simulink library "SimscapeCustomComponents_lib"  (R2025b)
settings: Solver=VariableStepAuto  StartTime=0.0  StopTime=10.0  RelTol=1e-3
undefined symbols (not defined in the file or in its folder): base, baseVdc, capacity, DiscIntNeverNeededParam, ee_sli_rtmsupport, filterInductance, freqeuncy, frequency, gcbh, gflInverter, gfmInverter, iMaxPU, Inertia, initialSOC, plantRating, solar, Ts, ups, Vac, windSystem, windTurbine
libraries: fl_lib x397, nesl_utility x171, eeGeneralControl x85, ee_lib x82, simulink x72, datacenter_lib x68, eeTransforms x38, slpidlib x24, buildingEnergy_lib x20, SimscapeFluids_lib x17, eeSinusoidalMeasurementV2 x8, eePwmGenerator x8
(part 2 of 24)

== system SimscapeCustomComponents_lib/Datacenter/CDU ==
  CDU (LUT) : Subsystem  mask{numPump=2, flowrate_vec=[100:100:1000]/60000, capacity_vec=10000*ones(1,10), effPump_vec=[0.4,0.42,0.45,0.5,0.55,0.6,0.62,0.65,0.65,0.64], prDrop_mat=1000*[0.28,1.11,2.5,4.44,6.94,10,13.61,17.78,22.5,27.78; 5.6,2.22,5,8.88,13.88,20,27.22,35.56,45,55.56]', speed=1}
      mask prompts: numPump "Total number of pumps (-)"; flowrate_vec "Coolant volumetric flowrate vector (m^3/s)"; capacity_vec "Heat exchanger capacity vector (W)"; effPump_vec "Pump efficiency vector, 0-1 (-)"; prDrop_mat "Pressure drop (Pa)"; speed "Pump speed scaling (-)"
      settings: CopyFcn=set_param(gcbh,'LinkStatus','none');  PortSchema="{\"entries\":[{\"content\":{\"sides\":[{\"content\":{\"connectorIds\":[\"LConn1\",\"LConn2\"]},\"type\":\"ConnectorPlacement.EquallySpacedRectSide\",\"uuid\":\"dd9276e8-a048-49df-a05c-f18b45aafce3\"},{\"content\":{\"connectorIds\":[\"RConn1\",\"RConn2\"],\"side\":\"RIGHT\"},\"type\":\"ConnectorPlacement.EquallySpacedRectSide\",\"uuid\":\"f4cbe01b-cfd4-4d60-aff7-a07955033ed5\"},{\"content\":{\"connectorIds\":[\"LConn3\"],\"side\":\"TOP\"},\"type\":\"ConnectorPlacement.EquallySpacedRectSide\",\"uuid\":\"ad27df56-4241-452c-8570-6a66062dd2f2\"}]},\"type\":\"ConnectorPlacement.EquallySpacedConnector\",\"uuid\":\"0333b5f9-1896-45e0-922d-790b0e5dd980\"}],\"packageUris\":[\"http://schema.mathworks.com/mf0/Connector/R2020b\"],\"version\":\"1.0\"}"
      mask Help: web("DocumentationCDULUT.html")
      mask DialogControl Container4 Prompt: CDU
      mask Display: image('icon_CDUtableBased.png');
  CDU (TL) : Subsystem  mask{extFluidMdot=[.3, .5, 1, 1.3, 1.7, 2, 2.6, 3.3], extFluidPrDrop=ones(1,8), extFluidVol=0.01, extFluidPipeArea=0.01, intFluidMdot=[.3, .5, .6, .7, 1, 1.4, 1.9, 2.3], intFluidPrDrop=ones(1,8), intFluidVol=0.01, intFluidPipeArea=0.01, spDissipationTbl=[.324, .3533, .404, .4253, .4333, .4373, .4453, .4533; .3813, .424, .496, .5307, .544, .5547, .5693, .5787; .4267, .4827, .5813, .6173, .6413, .6573, .672, .6827; .4613, .528, .64, .6987, .7267, .7467, .7707, .7853; .5533, .6467, .8227, .928, .9853, 1.0187, 1.0653, 1.0973; .58, .688, .8853, 1.0147, 1.08, 1.124, 1.176, 1.2147; .624, .7467, .992, 1.148, 1.244, 1.304, 1.3773, 1.4267; .656, .7907, 1.0667, 1.26, 1.376, 1.452, 1.548, 1.612], effPipeLen=5, pumpCapacityVec=[0.1:0.1:1.2]/998, pumpRefHeadVec=[239, 238.5, 232, 230, 222, 216, 208, 196, 186, 170,150,130], pumpRefBrkPowVec=[0.3,0.4,0.45,0.5,0.55,0.6,0.65,0.7,0.75,0.78,0.79,0.798], pumpEff=[20,40,50,60,65,70,75,75,75,73,68,60]/100, nPumps=3, speedLimFactor=1, pumpNominalRPM=3500, pumpImpellerDiaFactor=1, iniT=293, iniP=0.101325, refT=293, refP=0.101325, refDensity=998}
      mask prompts: extFluidMdot "External liquid loop mass flow rate vector (kg/s)"; extFluidPrDrop "External liquid loop pressure drop vector (kPa)"; extFluidVol "External liquid volume in heat exchanger (m^3)"; extFluidPipeArea "External liquid loop pipe cross-sectional area (m^2)"; intFluidMdot "Internal liquid loop mass flow rate vector (kg/s)"; intFluidPrDrop "Internal liquid loop pressure drop vector (kPa)"; intFluidVol "Internal liquid volume in heat exchanger (m^3)"; intFluidPipeArea "Internal liquid loop pipe cross-sectional area (m^2)"; spDissipationTbl "Specific dissipation table, SD[mdot_int,mdot_ext] (kW/K)"; effPipeLen "Effective pipe length for rack cooling (m)"; pumpCapacityVec "Reference capacity vector for each pump (m^3/s)"; pumpRefHeadVec "Reference head vector for each pump (m)"; pumpRefBrkPowVec "Reference brake power vector (kW)"; pumpEff "Electrical efficiency vector, 0-1 (-)"; nPumps "Total number of pumps (-)"; speedLimFactor "Pump speed upper limit factor (-)"; pumpNominalRPM "Pump nominal rating (rpm)"; pumpImpellerDiaFactor "Impeller diameter scale factor (-)"; iniT "Initial temperature (K)"; iniP "Initial pressure (MPa)"; refT "Reference flow temperature (K)"; refP "Reference flow pressure (MPa)"; refDensity "Reference density for internal liquid (kg/m^3)"
      settings: CopyFcn=set_param(gcbh,'LinkStatus','none');  PortSchema="{\"entries\":[{\"content\":{\"sides\":[{\"content\":{\"connectorIds\":[\"LConn1\",\"LConn2\",\"LConn3\"]},\"type\":\"ConnectorPlacement.EquallySpacedRectSide\",\"uuid\":\"dd9276e8-a048-49df-a05c-f18b45aafce3\"},{\"content\":{\"connectorIds\":[\"RConn1\",\"RConn2\"],\"side\":\"RIGHT\"},\"type\":\"ConnectorPlacement.EquallySpacedRectSide\",\"uuid\":\"f4cbe01b-cfd4-4d60-aff7-a07955033ed5\"},{\"content\":{\"connectorIds\":[\"LConn4\"],\"side\":\"TOP\"},\"type\":\"ConnectorPlacement.EquallySpacedRectSide\",\"uuid\":\"ad27df56-4241-452c-8570-6a66062dd2f2\"}]},\"type\":\"ConnectorPlacement.EquallySpacedConnector\",\"uuid\":\"0333b5f9-1896-45e0-922d-790b0e5dd980\"}],\"packageUris\":[\"http://schema.mathworks.com/mf0/Connector/R2020b\"],\"version\":\"1.0\"}"
      mask Help: web("DocumentationCDUTL.html")
      mask DialogControl Container5 Prompt: Heat Exchanger
      mask DialogControl Container8 Prompt: Set External Fluid Properties
      mask DialogControl Container7 Prompt: Set Internal Fluid Properties
      mask DialogControl Container9 Prompt: Heat Transfer
      mask DialogControl Container6 Prompt: Pumps
      mask DialogControl Container4 Prompt: Initial Conditions
      mask Display: image('icon_CDUthermalLiquid.png');
  CDU (TL) Detailed : Subsystem  mask{extFluidMdot=[.3, .5, 1, 1.3, 1.7, 2, 2.6, 3.3], extFluidPrDrop=ones(1,8), extFluidVol=0.01, extFluidPipeArea=0.01, intFluidMdot=[.3, .5, .6, .7, 1, 1.4, 1.9, 2.3], intFluidPrDrop=ones(1,8), intFluidVol=0.01, intFluidPipeArea=0.01, spDissipationTbl=[.324, .3533, .404, .4253, .4333, .4373, .4453, .4533; .3813, .424, .496, .5307, .544, .5547, .5693, .5787; .4267, .4827, .5813, .6173, .6413, .6573, .672, .6827; .4613, .528, .64, .6987, .7267, .7467, .7707, .7853; .5533, .6467, .8227, .928, .9853, 1.0187, 1.0653, 1.0973; .58, .688, .8853, 1.0147, 1.08, 1.124, 1.176, 1.2147; .624, .7467, .992, 1.148, 1.244, 1.304, 1.3773, 1.4267; .656, .7907, 1.0667, 1.26, 1.376, 1.452, 1.548, 1.612], pumpCapacityVec=[0.1:0.1:1.2]/998, pumpRefHeadVec=[239, 238.5, 232, 230, 222, 216, 208, 196, 186, 170,150,130], pumpRefBrkPowVec=[0.3,0.4,0.45,0.5,0.55,0.6,0.65,0.7,0.75,0.78,0.79,0.798], pumpEff=[20,40,50,60,65,70,75,75,75,73,68,60]/100, nPumps=3, speedLimFactor=1, pumpNominalRPM=3500, pumpImpellerDiaFactor=1, iniT=293, iniP=0.101325, refT=293, refP=0.101325, refDensity=998}
      mask prompts: extFluidMdot "External liquid loop mass flow rate vector (kg/s)"; extFluidPrDrop "External liquid loop pressure drop vector (kPa)"; extFluidVol "External liquid volume in heat exchanger (m^3)"; extFluidPipeArea "External liquid loop pipe cross-sectional area (m^2)"; intFluidMdot "Internal liquid loop mass flow rate vector (kg/s)"; intFluidPrDrop "Internal liquid loop pressure drop vector (kPa)"; intFluidVol "Internal liquid volume in heat exchanger (m^3)"; intFluidPipeArea "Internal liquid loop pipe cross-sectional area (m^2)"; spDissipationTbl "Specific dissipation table, SD[mdot_int,mdot_ext] (kW/K)"; pumpCapacityVec "Reference capacity vector for each pump (m^3/s)"; pumpRefHeadVec "Reference head vector for each pump (m)"; pumpRefBrkPowVec "Reference brake power vector (kW)"; pumpEff "Electrical efficiency vector, 0-1 (-)"; nPumps "Total number of pumps (-)"; speedLimFactor "Pump speed upper limit factor (-)"; pumpNominalRPM "Pump nominal rating (rpm)"; pumpImpellerDiaFactor "Impeller diameter scale factor (-)"; iniT "Initial temperature (K)"; iniP "Initial pressure (MPa)"; refT "Reference flow temperature (K)"; refP "Reference flow pressure (MPa)"; refDensity "Reference density for internal liquid (kg/m^3)"
      settings: CopyFcn=set_param(gcbh,'LinkStatus','none');  PortSchema="{\"entries\":[{\"content\":{\"sides\":[{\"content\":{\"connectorIds\":[\"LConn1\",\"LConn2\",\"LConn3\"]},\"type\":\"ConnectorPlacement.EquallySpacedRectSide\",\"uuid\":\"f1196858-c1c1-4a92-9579-b8bafb400d5a\"},{\"content\":{\"connectorIds\":[\"RConn1\",\"RConn2\"],\"side\":\"RIGHT\"},\"type\":\"ConnectorPlacement.EquallySpacedRectSide\",\"uuid\":\"0b2555b3-cd40-4e71-81ae-83eafd2a0952\"},{\"content\":{\"connectorIds\":[\"LConn4\",\"LConn5\"],\"side\":\"TOP\"},\"type\":\"ConnectorPlacement.EquallySpacedRectSide\",\"uuid\":\"202bfcad-adb5-4fb7-94c5-4d194a2e1d47\"}]},\"type\":\"ConnectorPlacement.EquallySpacedConnector\",\"uuid\":\"91782cfb-007a-4e62-9f99-de6082fc4e38\"}],\"packageUris\":[\"http://schema.mathworks.com/mf0/Connector/R2020b\"],\"version\":\"1.0\"}"
      mask Help: web("DocumentationCDUTL.html")
      mask DialogControl Container5 Prompt: Heat Exchanger
      mask DialogControl Container8 Prompt: Set External Fluid Properties
      mask DialogControl Container7 Prompt: Set Internal Fluid Properties
      mask DialogControl Container9 Prompt: Heat Transfer
      mask DialogControl Container6 Prompt: Pumps
      mask DialogControl Container4 Prompt: Initial Conditions
      mask Display: image('icon_CDUthermalLiquidDetailed.png');
  Rack Air Cooling : Subsystem  mask{nFans=5, flowVec=[0.1 0.2 0.3 0.4 0.5], prDropVec=[50 100 150 220 280], fanEffVec=[0.58, 0.60, 0.61, 0.60, 0.59], fluidDen=1.28, fluidCp=1005}
      mask prompts: nFans "Number of fans (-)"; flowVec "Fan flow rate vector (m^3/s)"; prDropVec "Pressure drop vector (Pa)"; fanEffVec "Fan efficiency vector (-)"; fluidDen "Fluid density (kg/m^3)"; fluidCp "Fluid heat capacity (J/(Kg*K))"
      settings: CopyFcn=set_param(gcbh,'LinkStatus','none');
      mask Help: web("DocumentationRackAirCooling.html")
      mask DialogControl Container3 Prompt: Fans
      mask DialogControl Container4 Prompt: Fluid Properties
      mask Display: image('icon_PDUfanCooling.png');

== system SimscapeCustomComponents_lib/Datacenter/Facilities ==
  CHB Module (Average Model) : datacenter_lib/CHB Module (Average Model)  OnResistance=1e-3 Ohm  GridVoltage=13800 V  TotalDCVoltage=13200 V  iAC_specify=off  iAC_priority=None  iAC=0 A  iAC_nominal_specify=off  iAC_nominal_value=1  iAC_nominal_unit=A  vAC_specify=off  vAC_priority=None  vAC=0 V  vAC_nominal_specify=off  vAC_nominal_value=1  vAC_nominal_unit=V  iDC_specify=off  iDC_priority=None  iDC=0 A  iDC_nominal_specify=off  iDC_nominal_value=1  iDC_nominal_unit=A  vDC_specify=off  vDC_priority=None  vDC=0 V  vDC_nominal_specify=off  vDC_nominal_value=1  vDC_nominal_unit=V  vOn_specify=off  vOn_priority=None  vOn=0 V  vOn_nominal_specify=off  vOn_nominal_value=1  vOn_nominal_unit=V
      settings: InternalSimscapePortConfiguration="{\"Bottom\":[],\"Left\":[{\"id\":\"m\",\"label\":\"m\",\"type\":\"input\"},{\"id\":\"ACPositive\",\"label\":\"AC+\",\"type\":\"foundation.electrical.electrical\"},{\"id\":\"ACNegative\",\"label\":\"AC-\",\"type\":\"foundation.electrical.electrical\"}],\"Right\":[{\"id\":\"DCPositive\",\"label\":\"DC+\",\"type\":\"foundation.electrical.electrical\"},{\"id\":\"DCNegative\",\"label\":\"DC-\",\"type\":\"foundation.electrical.electrical\"}],\"Top\":[]}"
  CHB Phase Leg (Average Model) : datacenter_lib/CHB Phase Leg (Average Model)  NumModules=3  OnResistance=1e-3 Ohm  InitialDCVoltage=4400 V  GridVoltage=13800 V  TotalDCVoltage=13200 V
      settings: InternalSimscapePortConfiguration="{\"Bottom\":[],\"Left\":[{\"id\":\"ACPositive\",\"label\":\"AC+\",\"type\":\"foundation.electrical.electrical\"},{\"id\":\"ACNegative\",\"label\":\"AC-\",\"type\":\"foundation.electrical.electrical\"},{\"id\":\"m\",\"label\":\"m\",\"type\":\"input\"}],\"Right\":[{\"id\":\"DCPositive\",\"label\":\"DC+\",\"type\":\"foundation.electrical.electrical\"},{\"id\":\"DCNegative\",\"label\":\"DC-\",\"type\":\"foundation.electrical.electrical\"}],\"Top\":[]}"
  Chiller : Subsystem  mask{nominalRating=270, nominalFlowrate=185, nominalPrDrop=0.05, cop=13, volume=1, portArea=0.01, initialP=0.101325, initialT=300}
      mask prompts: nominalRating "Nominal rating (kW)"; nominalFlowrate "Nominal flowrate (kg/s)"; nominalPrDrop "Nominal pressure drop (MPa)"; cop "Coefficient of performance (-)"; volume "Chiller volume (m^3)"; portArea "Cross-sectional port area (m^2)"; initialP "Initial pressure (MPa)"; initialT "Initial temperature (K)"
      settings: CopyFcn=set_param(gcbh,'LinkStatus','none');  PortSchema="{\"entries\":[{\"content\":{\"sides\":[{\"content\":{\"connectorIds\":[\"LConn1\",\"LConn2\"]},\"type\":\"ConnectorPlacement.EquallySpacedRectSide\",\"uuid\":\"7d4232d9-e275-4255-9dc4-bc3f1c69ec46\"},{\"content\":{\"connectorIds\":[\"RConn1\",\"RConn2\"],\"side\":\"RIGHT\"},\"type\":\"ConnectorPlacement.EquallySpacedRectSide\",\"uuid\":\"7ca0ea83-7974-4453-97b6-22bfcf77b4f1\"},{\"content\":{\"connectorIds\":[\"LConn3\",\"LConn4\"],\"side\":\"TOP\"},\"type\":\"ConnectorPlacement.EquallySpacedRectSide\",\"uuid\":\"65c43657-b3f1-43d9-9625-8376acff2e22\"},{\"content\":{\"side\":\"BOTTOM\"},\"type\":\"ConnectorPlacement.EquallySpacedRectSide\",\"uuid\":\"1eb88563-12e2-4927-be7c-afaa658f242e\"}]},\"type\":\"ConnectorPlacement.EquallySpacedConnector\",\"uuid\":\"9af448fb-8903-42ba-af4c-44d5135333f1\"}],\"packageUris\":[\"http://schema.mathworks.com/mf0/Connector/R2020b\"],\"version\":\"1.0\"}"
      mask Help: web('DocumentationChiller.html')
      mask DialogControl Container2 Prompt: Rating
      mask DialogControl Container3 Prompt: Initial Conditions
      mask Display: image('icon_Chiller.png');
  Compute Profile Source (LLM Workload Generator) : datacenter_lib/Compute Profile Source (LLM Workload Generator)  gpuModel=GPUModel.B200  numGPUs=288  workloadType=WorkloadType.Training  timeScale=1  tokenSource=TokenSource.Fixed  showAdvanced=false  customPeakTFLOPS=1000  customHbmBW=4e12 1/s  hbmBW=8e12 1/s  interNodeBW=50e9 1/s  llmSize=LLMModelSize.Llama_70B  customNumParams_B=70  customNumLayers=80  customPrecision=2  parallelism=ParallelismStrategy.TP8_PP4  customTP=8  customPP=4  microBatch=8  globalBatch=2048  seqLength=2048  idleUtil=0.05  fwdUtil=0.85  bwdUtil=0.92  commSyncUtil=0.15  prompt_tokens=512  output_tokens=256  num_concurrent=8  batch_size=8  allreduce_latency=5e-6 s  baseInfUtil=0.08  baseInfFrac=0.10  MFU=0.85  checkpointOverhead=0.03  stragglerOverhead=0.02  trainableParamFrac=0.02  evalInterval=5  evalBatches=2  ft_checkpointOverhead=0.05  enableNoise=true  noiseAmplitude=0.08  stepJitter=0.15  enableFilter=false  filterTimeConstant=0.01 s  t_step_specify=off  t_step_priority=Low  t_step=0 s  t_step_nominal_specify=off  t_step_nominal_value=1  t_step_nominal_unit=s  phase_id_specify=off  phase_id_priority=None  phase_id=0  phase_id_nominal_specify=off  phase_id_nominal_value=1  phase_id_nominal_unit=1  utilization_specify=off  utilization_priority=None  utilization=0  utilization_nominal_specify=off  utilization_nominal_value=1  utilization_nominal_unit=1  step_count_specify=off  step_count_priority=None  step_count=0  step_count_nominal_specify=off  step_count_nominal_value=1  step_count_nominal_unit=1  tc_utilization_specify=off  tc_utilization_priority=None  tc_utilization=0  tc_utilization_nominal_specify=off  tc_utilization_nominal_value=1  tc_utilization_nominal_unit=1  hbm_utilization_specify=off  hbm_utilization_priority=None  hbm_utilization=0  hbm_utilization_nominal_specify=off  hbm_utilization_nominal_value=1  hbm_utilization_nominal_unit=1  tokens_per_sec_obs_specify=off  tokens_per_sec_obs_priority=None  tokens_per_sec_obs=0 1/s  tokens_per_sec_obs_nominal_specify=off  tokens_per_sec_obs_nominal_value=1  tokens_per_sec_obs_nominal_unit=1/s  ttft_obs_specify=off  ttft_obs_priority=None  ttft_obs=0 s  ttft_obs_nominal_specify=off  ttft_obs_nominal_value=1  ttft_obs_nominal_unit=s
      settings: InternalSimscapePortConfiguration="{\"Bottom\":[],\"Left\":[{\"id\":\"prompt_len_in\",\"label\":\"Tn(in)\",\"type\":\"input\"}],\"Right\":[{\"id\":\"compute\",\"label\":\"C\",\"type\":\"output\"},{\"id\":\"U\",\"label\":\"U\",\"type\":\"output\"}],\"Top\":[]}"
  DAB Generalized Average Model : datacenter_lib/DAB Generalized Average Model  N=1  L1=68.2e-6 H  L2=68.2e-6 H  Rt=0.5 Ohm  Co=540e-6 F  fs=10000 Hz  vo0_init=0 V  it1R_init=0 A  it1I_init=0 A  include_esr=false  Rc=0.25 Ohm  i_in_specify=off  i_in_priority=None  i_in=0 A  i_in_nominal_specify=off  i_in_nominal_value=1  i_in_nominal_unit=A  i_out_specify=off  i_out_priority=None  i_out=0 A  i_out_nominal_specify=off  i_out_nominal_value=1  i_out_nominal_unit=A  v_in_specify=off  v_in_priority=None  v_in=0 V  v_in_nominal_specify=off  v_in_nominal_value=1  v_in_nominal_unit=V  v_out_specify=off  v_out_priority=None  v_out=0 V  v_out_nominal_specify=off  v_out_nominal_value=1  v_out_nominal_unit=V
      settings: InternalSimscapePortConfiguration="{\"Bottom\":[],\"Left\":[{\"id\":\"p_in\",\"label\":\"V+\",\"type\":\"foundation.electrical.electrical\"},{\"id\":\"n_in\",\"label\":\"V-\",\"type\":\"foundation.electrical.electrical\"},{\"id\":\"d\",\"label\":\"d\",\"type\":\"input\"}],\"Right\":[{\"id\":\"p_out\",\"label\":\"Vo+\",\"type\":\"foundation.electrical.electrical\"},{\"id\":\"n_out\",\"label\":\"Vo-\",\"type\":\"foundation.electrical.electrical\"}],\"Top\":[]}"
  PSU PFC Stage (Average Model) : datacenter_lib/PSU PFC Stage (Average Model)  C_dc=2e-3 F  V_dc_ref=400 V  Kp_pfc=1.0 W/V  Ki_pfc=60 W/(V*s)  eta_pfc=0.97  P_max=130000 W  G_damp=0.02 1/Ohm  tau_rms=0.040 s  V_nom=277 V  L_ac=0.5e-3 H  R_ac=0.01 Ohm  i_ac_specify=off  i_ac_priority=None  i_ac=0 A  i_ac_nominal_specify=off  i_ac_nominal_value=1  i_ac_nominal_unit=A  v_ac_specify=off  v_ac_priority=Low  v_ac=277 V  v_ac_nominal_specify=off  v_ac_nominal_value=1  v_ac_nominal_unit=V  v_dc_specify=off  v_dc_priority=High  v_dc=400 V  v_dc_nominal_specify=off  v_dc_nominal_value=1  v_dc_nominal_unit=V  i_dc_specify=off  i_dc_priority=None  i_dc=0 A  i_dc_nominal_specify=off  i_dc_nominal_value=1  i_dc_nominal_unit=A  pfc_integrator_specify=off  pfc_integrator_priority=None  pfc_integrator=0 V*s  pfc_integrator_nominal_specify=off  pfc_integrator_nominal_value=1  pfc_integrator_nominal_unit=V*s  v_rms_sq_specify=off  v_rms_sq_priority=Low  v_rms_sq=76729 V^2  v_rms_sq_nominal_specify=off  v_rms_sq_nominal_value=1  v_rms_sq_nominal_unit=V^2
      settings: InternalSimscapePortConfiguration="{\"Bottom\":[],\"Left\":[{\"id\":\"p\",\"label\":\"AC+\",\"type\":\"foundation.electrical.electrical\"},{\"id\":\"n\",\"label\":\"AC-\",\"type\":\"foundation.electrical.electrical\"}],\"Right\":[{\"id\":\"dc_p\",\"label\":\"DC+\",\"type\":\"foundation.electrical.electrical\"},{\"id\":\"dc_n\",\"label\":\"DC-\",\"type\":\"foundation.electrical.electrical\"}],\"Top\":[]}"
  Solid State Transformer : Subsystem  mask(Solid State Transformer){inputVoltage=13800, dcBusVoltage=4400, dcOutputVoltage=800, frequency=60, numModules=3, Kp_dab=5.5, Ki_dab=130, dab_sat_upper=0.45, dab_sat_lower=-0.45, dcBusCapacitance=0.005, filterInductance=0.01, filterResistance=0.1, dab_sampleTime=5e-05, Vdc_init=4400}
      mask prompts: inputVoltage "Input Voltage - Phase to Phase RMS (V)"; dcBusVoltage "DC Bus Voltage per Module (V)"; dcOutputVoltage "DC Output Voltage (V)"; frequency "Grid Frequency (Hz)"; numModules "Number of CHB Modules per Phase"; Kp_dab "Proportional Gain (Kp)"; Ki_dab "Integral Gain (Ki)"; dab_sat_upper "Phase Shift Upper Limit"; dab_sat_lower "Phase Shift Lower Limit"; dcBusCapacitance "DC Bus Capacitance (F)"; filterInductance "Filter Inductance (H)"; filterResistance "Filter Resistance (Ohm)"; dab_sampleTime "DAB sample time (s)"; Vdc_init "Initial DC bus voltage (V)"
      mask help: Solid State Transformer with CHB rectifier and DAB DC-DC converters. Three-phase input, isolated DC output.
      mask init:
      | % SST Mask Initialization
      | % Propagate DAB PI gains to all 9 DAB controllers
      | phases = {'Subsystem1', 'Subsystem2', 'Subsystem3'};
      | 
      | % Support per-phase capacitance: scalar or [Ca Cb Cc] vector
      | if isscalar(dcBusCapacitance)
      |     capPerPhase = dcBusCapacitance * [1 1 1];
      | else
      |     capPerPhase = dcBusCapacitance;
      | end
      | 
      | % Support per-phase initial voltage: scalar or [Va Vb Vc] vector
      | if isscalar(Vdc_init)
      |     vInitPerPhase = Vdc_init * [1 1 1];
      | else
      |     vInitPerPhase = Vdc_init;
      | end
      | 
      | for p = 1:3
      |     % Propagate DC bus capacitance (per-phase)
      |     caps = {'Capacitor', 'Capacitor1', 'Capacitor2'};
      |     for c = 1:3
      |         capPath = [gcb, '/Converters/', phases{p}, '/', caps{c}];
      |         set_param(capPath, 'c', num2str(capPerPhase(p)));
      |         set_param(capPath, 'vc', num2str(vInitPerPhase(p)));
      |     end
      | end
      | 
      | % Propagate filter parameters
      | rlPath = [gcb, '/Filter & AC measurements/RL filter'];
      | set_param(rlPath, 'L', num2str(filterInductance));
      | set_param(rlPath, 'R', num2str(filterResistance));
      settings: CopyFcn=set_param(gcbh,'LinkStatus','none');
      mask Help: web("DocumentationSolidStateTransformer.html")
      mask DialogControl GeneralTab Prompt: General
      mask DialogControl PFCControlTab Prompt: PFC Control
      mask DialogControl openPFCController Prompt: Edit PFC Controller
      mask DialogControl openPFCController Callback:
      | blockPath = [gcb,'/PFC Rectifier Controller'];
      | open_system(blockPath, 'mask');
      mask DialogControl HBridgeTab Prompt: H-Bridge
      mask DialogControl openCHBBlock Prompt: Edit CHB Phase Leg Parameters
      mask DialogControl openCHBBlock Callback:
      | blockPath = [gcb,'/Converters/Subsystem1/CHB Phase Leg' char(10) '(Average Model)'];
      | open_system(blockPath, 'mask');
      mask DialogControl DABTab Prompt: DAB
      mask DialogControl openDABBlock Prompt: Edit DAB Parameters
      mask DialogControl openDABBlock Callback:
      | blockPath = [gcb,'/Converters/Subsystem1/DAB Generalized' char(10) 'Average Model'];
      | open_system(blockPath, 'mask');
      mask Display: image('sst_icon.svg')

== system SimscapeCustomComponents_lib/Datacenter/PDU ==
  Cold Plate : Subsystem  mask{pipeLen=1, pipeArea=1e-3, pipeDia=5e-3, pipeLenXtra=1e-1, thermalR=1e-2, initialT=293, initialP=0.101325}
      mask prompts: pipeLen "Cold plate pipe length (m)"; pipeArea "Pipe cross-section area (m^2)"; pipeDia "Pipe hydraulic diameter (m)"; pipeLenXtra "Aggregate equivalent length of local resistances (m)"; thermalR "IT tray to cold plate thermal resistance (K/W)"; initialT "Initial temperature (K)"; initialP "Initial pressure (MPa)"
      settings: CopyFcn=set_param(gcbh,'LinkStatus','none');  PortSchema="{\"entries\":[{\"content\":{\"sides\":[{\"content\":{\"connectorIds\":[\"LConn1\"]},\"type\":\"ConnectorPlacement.EquallySpacedRectSide\",\"uuid\":\"8838d57f-01eb-4279-bd1c-25d25bcf5ace\"},{\"content\":{\"connectorIds\":[\"RConn1\"],\"side\":\"RIGHT\"},\"type\":\"ConnectorPlacement.EquallySpacedRectSide\",\"uuid\":\"56ae8252-1580-44dd-87b9-8c427bc34f49\"},{\"content\":{\"connectorIds\":[\"LConn2\"],\"side\":\"TOP\"},\"type\":\"ConnectorPlacement.EquallySpacedRectSide\",\"uuid\":\"52c6abaa-a3e9-4948-a21c-7378e8bd6fd9\"}]},\"type\":\"ConnectorPlacement.EquallySpacedConnector\",\"uuid\":\"7eb709cb-ec6a-4cc7-adbc-64cff18012b9\"}],\"packageUris\":[\"http://schema.mathworks.com/mf0/Connector/R2020b\"],\"version\":\"1.0\"}"
      mask Help: web("DocumentationColdPlate.html")
      mask DialogControl Container4 Prompt: Cold Plate
      mask DialogControl Container5 Prompt: Initial Conditions
      mask Display: image('icon_coldplate.png');
  PDU Racks : Subsystem  mask{nTrays=6, nRacks=4, trayMass=5, trayCp=2000, trayThermalR=0.1, nGPU=1, gpuTDPperDie=1200, gpuIdlePower=300, gpuHBMpower=80, gpuExponent=1.4, gpuHBMutil=0.7, gpuLeakage=1.5, gpuNominalDieT=350, gpuDieThermalC=50, gpuHeatSinkR=0.15, gpuSurfArea=0.01, gpuAmbientR=0.5, nCPU=1, cpuTDPperSocket=350, cpuIdlePower=80, cpuExponent=1.1, cpuLeakage=1.5, cpuNominalDieT=350, cpuDieThermalC=50, cpuHeatSinkR=0.15, cpuSurfArea=0.01, cpuAmbientR=0.5, initialT=350, htc=10}
      mask prompts: nTrays "Number of IT trays per rack (-)"; nRacks "Number of racks (-)"; trayMass "Tray mass (kg)"; trayCp "Tray specific heat capacity (J/kg*K)"; trayThermalR "Tray to external thermal resistance (K/W)"; nGPU "Number of GPU per tray (-)"; gpuTDPperDie "GPU TDP per die (W)"; gpuIdlePower "GPU idle power (W)"; gpuHBMpower "HBM power per GPU (W)"; gpuExponent "GPU power utilization exponent (-)"; gpuHBMutil "HBM utilization as fraction of compute utilization (-)"; gpuLeakage "Leakage increase per K above nominal temperature (W/K)"; gpuNominalDieT "Nominal die temperature at TDP (K)"; gpuDieThermalC "GPU die thermal capacitance (J/K)"; gpuHeatSinkR "GPU die-heat-sink thermal resistance (K/W)"; gpuSurfArea "Surface area per die for ambient heat transfer (m^2)"; gpuAmbientR "GPU die-ambient thermal resistance (K/W)"; nCPU "Number of CPU per tray (-)"; cpuTDPperSocket "CPU TDP per socket (W)"; cpuIdlePower "CPU idle power per socket (W)"; cpuExponent "CPU power utilization exponent (-)"; cpuLeakage "Leakage increase per K above nominal temperature (W/K)"; cpuNominalDieT "Nominal die temperature at TDP (K)"; cpuDieThermalC "CPU die thermal capacitance (J/K)"; cpuHeatSinkR "CPU die-heat-sink thermal resistance (K/W)"; cpuSurfArea "Surface area per die for ambient heat transfer (m^2)"; cpuAmbientR "CPU die-ambient thermal resistance (K/W)"; initialT "Initial temperature (K)"; htc "Heat transfer coefficient to ambient (W/m^2.K)"
      settings: CopyFcn=set_param(gcbh,'LinkStatus','none');  PortSchema="{\"entries\":[{\"content\":{\"sides\":[{\"content\":{\"connectorIds\":[\"LConn1\",\"LConn2\",\"LConn3\"]},\"type\":\"ConnectorPlacement.EquallySpacedRectSide\",\"uuid\":\"1a9a884a-dab1-4495-bf62-c6b2de6c1039\"},{\"content\":{\"connectorIds\":[\"RConn1\",\"RConn2\",\"RConn3\"],\"side\":\"RIGHT\"},\"type\":\"ConnectorPlacement.EquallySpacedRectSide\",\"uuid\":\"05c53434-51c1-4fee-b885-c321dcda8b6b\"},{\"content\":{\"side\":\"TOP\"},\"type\":\"ConnectorPlacement.EquallySpacedRectSide\",\"uuid\":\"c7b5c534-d596-4858-a133-27f005e6c9d4\"},{\"content\":{\"connectorIds\":[\"RConn4\"],\"side\":\"BOTTOM\"},\"type\":\"ConnectorPlacement.EquallySpacedRectSide\",\"uuid\":\"693f3c99-4296-4d86-bfcc-da753d3e576f\"}]},\"type\":\"ConnectorPlacement.EquallySpacedConnector\",\"uuid\":\"ed91c467-c4d0-403f-af16-bac0257594fd\"}],\"packageUris\":[\"http://schema.mathworks.com/mf0/Connector/R2020b\"],\"version\":\"1.0\"}"
      mask Help: web("DocumentationPDURacks.html")
      mask DialogControl Container10 Prompt: PDU Racks
      mask DialogControl getRatingButton Prompt: Get Rating
      mask DialogControl Container9 Prompt: IT Tray
      mask DialogControl Container6 Prompt: GPU
      mask DialogControl Container7 Prompt: CPU
      mask DialogControl Container8 Prompt: Initial Conditions
      mask Display: image('icon_PDURacks.png');
  PDU Racks (TL) : Subsystem  mask{nTrays=6, nRacks=4, trayMass=5, trayCp=2000, trayThermalR=0.1, pipeLen=1, pipeArea=1e-3, pipeDia=5e-3, pipeLenXtra=0.05, thermalKtc=0.01, nGPU=1, gpuTDPperDie=1200, gpuIdlePower=300, gpuHBMpower=80, gpuExponent=1.4, gpuHBMutil=0.7, gpuLeakage=1.5, gpuNominalDieT=350, gpuDieThermalC=50, gpuHeatSinkR=0.15, gpuSurfArea=0.01, gpuAmbientR=0.5, nCPU=1, cpuTDPperSocket=350, cpuIdlePower=80, cpuExponent=1.1, cpuLeakage=1.5, cpuNominalDieT=350, cpuDieThermalC=50, cpuHeatSinkR=0.15, cpuSurfArea=0.01, cpuAmbientR=0.5, initialT=350, initialP=0.101325, htc=10}
      mask prompts: nTrays "Number of IT trays per rack (-)"; nRacks "Number of racks (-)"; trayMass "Tray mass (kg)"; trayCp "Tray specific heat capacity (J/kg*K)"; trayThermalR "Tray to external thermal resistance (K/W)"; pipeLen "Cold plate pipe length (m)"; pipeArea "Cold plate pipe cross-sectional area (m^2)"; pipeDia "Cold plate pipe hydraulic diameter (m)"; pipeLenXtra "Cold plate pipe aggregate equivalent length of local resistances (m)"; thermalKtc "Tray to cold plate thermal resistance (K/W)"; nGPU "Number of GPU per tray (-)"; gpuTDPperDie "GPU TDP per die (W)"; gpuIdlePower "GPU idle power (W)"; gpuHBMpower "HBM power per GPU (W)"; gpuExponent "GPU power utilization exponent (-)"; gpuHBMutil "HBM utilization as fraction of compute utilization (-)"; gpuLeakage "Leakage increase per K above nominal temperature (W/K)"; gpuNominalDieT "Nominal die temperature at TDP (K)"; gpuDieThermalC "GPU die thermal capacitance (J/K)"; gpuHeatSinkR "GPU die-heat-sink thermal resistance (K/W)"; gpuSurfArea "Surface area per die for ambient heat transfer (m^2)"; gpuAmbientR "GPU die-ambient thermal resistance (K/W)"; nCPU "Number of CPU per tray (-)"; cpuTDPperSocket "CPU TDP per socket (W)"; cpuIdlePower "CPU idle power per socket (W)"; cpuExponent "CPU power utilization exponent (-)"; cpuLeakage "Leakage increase per K above nominal temperature (W/K)"; cpuNominalDieT "Nominal die temperature at TDP (K)"; cpuDieThermalC "CPU die thermal capacitance (J/K)"; cpuHeatSinkR "CPU die-heat-sink thermal resistance (K/W)"; cpuSurfArea "Surface area per die for ambient heat transfer (m^2)"; cpuAmbientR "CPU die-ambient thermal resistance (K/W)"; initialT "Initial temperature (K)"; initialP "Initial pressure (MPa)"; htc "Heat transfer coefficient to ambient (W/m^2.K)"
      settings: CopyFcn=set_param(gcbh,'LinkStatus','none');  PortSchema="{\"entries\":[{\"content\":{\"sides\":[{\"content\":{\"connectorIds\":[\"LConn1\",\"LConn2\",\"LConn3\"]},\"type\":\"ConnectorPlacement.EquallySpacedRectSide\",\"uuid\":\"39cab6a2-c76f-43a0-9a61-57ffbd8863b1\"},{\"content\":{\"connectorIds\":[\"RConn1\",\"RConn2\",\"RConn3\"],\"side\":\"RIGHT\"},\"type\":\"ConnectorPlacement.EquallySpacedRectSide\",\"uuid\":\"8dbc310f-d80c-499d-a8e3-7ab6fed33056\"},{\"content\":{\"side\":\"TOP\"},\"type\":\"ConnectorPlacement.EquallySpacedRectSide\",\"uuid\":\"edeccc9d-eefc-49d3-8062-c5510820acf3\"},{\"content\":{\"connectorIds\":[\"RConn4\",\"RConn5\"],\"side\":\"BOTTOM\"},\"type\":\"ConnectorPlacement.EquallySpacedRectSide\",\"uuid\":\"2bb1883a-38ad-4153-b5a2-578f43360854\"}]},\"type\":\"ConnectorPlacement.EquallySpacedConnector\",\"uuid\":\"59ce167c-b40d-422d-b962-f18524a07abd\"}],\"packageUris\":[\"http://schema.mathworks.com/mf0/Connector/R2020b\"],\"version\":\"1.0\"}"
      mask Help: web("DocumentationPDURacksTL.html")
      mask DialogControl Container10 Prompt: PDU Racks
      mask DialogControl getRatingButton Prompt: Get Rating
      mask DialogControl Container9 Prompt: IT Tray
      mask DialogControl Container6 Prompt: GPU
      mask DialogControl Container7 Prompt: CPU
      mask DialogControl Container8 Prompt: Initial Conditions
      mask Display: image('icon_PDURacksTL.png');
  Server Chip : datacenter_lib/Server Chip  processorType=ProcessorType.GPU  numGPUs=4  numCPUs=2  gpuTDP=1200 W  gpuIdlePower=300 W  gpuPowerExponent=1.4  hbmPowPerGPU=80 W  hbmUtilizationFrac=0.7  cpuTDP=350 W  cpuIdlePower=80 W  cpuPowerExponent=1.1  PleakageCoeff=1.5 W/K  chipTnominal=350 K  chipCth=50 J/K  T_specify=off  T_priority=High  T=350 K  T_nominal_specify=off  T_nominal_value=1  T_nominal_unit=K  Q_specify=off  Q_priority=None  Q=0 W  Q_nominal_specify=off  Q_nominal_value=1  Q_nominal_unit=W
      settings: InternalSimscapePortConfiguration="{\"Bottom\":[{\"id\":\"H\",\"label\":\"H\",\"type\":\"foundation.thermal.thermal\"}],\"Left\":[{\"id\":\"U\",\"label\":\"U\",\"type\":\"input\"}],\"Right\":[{\"id\":\"Pow\",\"label\":\"P\",\"type\":\"output\"},{\"id\":\"Tchip\",\"label\":\"T\",\"type\":\"output\"}],\"Top\":[]}"
  Server Tray : Subsystem  mask{nGPU=1, gpuTDPperDie=1200, gpuIdlePower=300, gpuHBMpower=80, gpuExponent=1.4, gpuHBMutil=0.7, gpuLeakage=1.5, gpuNominalDieT=350, gpuDieThermalC=50, gpuHeatSinkR=0.15, gpuSurfArea=0.01, gpuAmbientR=0.5, nCPU=1, cpuTDPperSocket=350, cpuIdlePower=80, cpuExponent=1.1, cpuLeakage=1.5, cpuNominalDieT=350, cpuDieThermalC=50, cpuHeatSinkR=0.15, cpuSurfArea=0.01, cpuAmbientR=0.5, trayMass=5, trayCp=2000, trayThermalR=0.1, initialT=350, htc=10}
      mask prompts: nGPU "Number of GPU (-)"; gpuTDPperDie "GPU TDP per die (W)"; gpuIdlePower "GPU idle power (W)"; gpuHBMpower "HBM power per GPU (W)"; gpuExponent "GPU power utilization exponent (-)"; gpuHBMutil "HBM utilization as fraction of compute utilization (-)"; gpuLeakage "Leakage increase per K above nominal temperature (W/K)"; gpuNominalDieT "Nominal die temperature at TDP (K)"; gpuDieThermalC "GPU die thermal capacitance (J/K)"; gpuHeatSinkR "GPU die-heat-sink thermal resistance (K/W)"; gpuSurfArea "Surface area per die for ambient heat transfer (m^2)"; gpuAmbientR "GPU die-ambient thermal resistance (K/W)"; nCPU "Number of CPU (-)"; cpuTDPperSocket "CPU TDP per socket (W)"; cpuIdlePower "CPU idle power per socket (W)"; cpuExponent "CPU power utilization exponent (-)"; cpuLeakage "Leakage increase per K above nominal temperature (W/K)"; cpuNominalDieT "Nominal die temperature at TDP (K)"; cpuDieThermalC "CPU die thermal capacitance (J/K)"; cpuHeatSinkR "CPU die-heat-sink thermal resistance (K/W)"; cpuSurfArea "Surface area per die for ambient heat transfer (m^2)"; cpuAmbientR "CPU die-ambient thermal resistance (K/W)"; trayMass "Tray mass (kg)"; trayCp "Tray specific heat capacity (J/kg*K)"; trayThermalR "Tray to external thermal resistance (K/W)"; initialT "Initial temperature (K)"; htc "Heat transfer coefficient to ambient (W/m^2.K)"
      settings: CopyFcn=set_param(gcbh,'LinkStatus','none');  PortSchema="{\"entries\":[{\"content\":{\"sides\":[{\"content\":{\"connectorIds\":[\"LConn1\",\"LConn2\",\"LConn3\"]},\"type\":\"ConnectorPlacement.EquallySpacedRectSide\",\"uuid\":\"893f21b9-92d6-433a-96e5-f8193a696c29\"},{\"content\":{\"connectorIds\":[\"RConn1\",\"RConn2\",\"RConn3\"],\"side\":\"RIGHT\"},\"type\":\"ConnectorPlacement.EquallySpacedRectSide\",\"uuid\":\"efd10409-70d8-4a6a-97a2-13f0e6f538e3\"},{\"content\":{\"side\":\"TOP\"},\"type\":\"ConnectorPlacement.EquallySpacedRectSide\",\"uuid\":\"8c9765cd-90e6-46de-916c-606bbb93143e\"},{\"content\":{\"connectorIds\":[\"RConn4\"],\"side\":\"BOTTOM\"},\"type\":\"ConnectorPlacement.EquallySpacedRectSide\",\"uuid\":\"9656b44e-d582-43b0-a7fe-c629821d6c27\"}]},\"type\":\"ConnectorPlacement.EquallySpacedConnector\",\"uuid\":\"add7a682-eb4b-4f46-a5b9-e161ccf96de5\"}],\"packageUris\":[\"http://schema.mathworks.com/mf0/Connector/R2020b\"],\"version\":\"1.0\"}"
      mask Help: web("DocumentationServerTray.html")
      mask DialogControl Container6 Prompt: GPU
      mask DialogControl Container7 Prompt: CPU
      mask DialogControl Container9 Prompt: IT Tray
      mask DialogControl Container8 Prompt: Initial Conditions
      mask Display: image('icon_serverPlate.png');
  Server Tray (TL) : Subsystem  mask{nGPU=1, gpuTDPperDie=1200, gpuIdlePower=300, gpuHBMpower=80, gpuExponent=1.4, gpuHBMutil=0.7, gpuLeakage=1.5, gpuNominalDieT=350, gpuDieThermalC=50, gpuHeatSinkR=0.15, gpuSurfArea=0.01, gpuAmbientR=0.5, nCPU=1, cpuTDPperSocket=350, cpuIdlePower=80, cpuExponent=1.1, cpuLeakage=1.5, cpuNominalDieT=350, cpuDieThermalC=50, cpuHeatSinkR=0.15, cpuSurfArea=0.01, cpuAmbientR=0.5, trayMass=5, trayCp=2000, trayThermalR=0.1, pipeLen=1, pipeArea=1e-3, pipeDia=5e-3, pipeLenXtra=0.05, thermalKtc=0.01, initialT=350, initialP=0.101325, htc=10}
      mask prompts: nGPU "Number of GPU (-)"; gpuTDPperDie "GPU TDP per die (W)"; gpuIdlePower "GPU idle power (W)"; gpuHBMpower "HBM power per GPU (W)"; gpuExponent "GPU power utilization exponent (-)"; gpuHBMutil "HBM utilization as fraction of compute utilization (-)"; gpuLeakage "Leakage increase per K above nominal temperature (W/K)"; gpuNominalDieT "Nominal die temperature at TDP (K)"; gpuDieThermalC "GPU die thermal capacitance (J/K)"; gpuHeatSinkR "GPU die-heat-sink thermal resistance (K/W)"; gpuSurfArea "Surface area per die for ambient heat transfer (m^2)"; gpuAmbientR "GPU die-ambient thermal resistance (K/W)"; nCPU "Number of CPU (-)"; cpuTDPperSocket "CPU TDP per socket (W)"; cpuIdlePower "CPU idle power per socket (W)"; cpuExponent "CPU power utilization exponent (-)"; cpuLeakage "Leakage increase per K above nominal temperature (W/K)"; cpuNominalDieT "Nominal die temperature at TDP (K)"; cpuDieThermalC "CPU die thermal capacitance (J/K)"; cpuHeatSinkR "CPU die-heat-sink thermal resistance (K/W)"; cpuSurfArea "Surface area per die for ambient heat transfer (m^2)"; cpuAmbientR "CPU die-ambient thermal resistance (K/W)"; trayMass "Tray mass (kg)"; trayCp "Tray specific heat capacity (J/kg*K)"; trayThermalR "Tray to external thermal resistance (K/W)"; pipeLen "Cold plate pipe length (m)"; pipeArea "Cold plate pipe cross-sectional area (m^2)"; pipeDia "Cold plate pipe hydraulic diameter (m)"; pipeLenXtra "Cold plate pipe aggregate equivalent length of local resistances (m)"; thermalKtc "Tray to cold plate thermal resistance (K/W)"; initialT "Initial temperature (K)"; initialP "Initial pressure (MPa)"; htc "Heat transfer coefficient to ambient (W/m^2.K)"
      settings: CopyFcn=set_param(gcbh,'LinkStatus','none');  PortSchema="{\"entries\":[{\"content\":{\"sides\":[{\"content\":{\"connectorIds\":[\"LConn1\",\"LConn2\",\"LConn3\"]},\"type\":\"ConnectorPlacement.EquallySpacedRectSide\",\"uuid\":\"d077d73c-67b3-4833-87c7-90e0b4257578\"},{\"content\":{\"connectorIds\":[\"RConn1\",\"RConn2\",\"RConn3\"],\"side\":\"RIGHT\"},\"type\":\"ConnectorPlacement.EquallySpacedRectSide\",\"uuid\":\"5339be23-611e-4862-9a5e-dd4e1a595af9\"},{\"content\":{\"side\":\"TOP\"},\"type\":\"ConnectorPlacement.EquallySpacedRectSide\",\"uuid\":\"df4f00c7-722c-4787-b527-29bc4d99befa\"},{\"content\":{\"connectorIds\":[\"RConn4\",\"RConn5\"],\"side\":\"BOTTOM\"},\"type\":\"ConnectorPlacement.EquallySpacedRectSide\",\"uuid\":\"45f86463-19b5-41c3-bb79-cbbcfbdd4a59\"}]},\"type\":\"ConnectorPlacement.EquallySpacedConnector\",\"uuid\":\"da9ddc4c-7978-4ef3-ba33-dfd55a606f60\"}],\"packageUris\":[\"http://schema.mathworks.com/mf0/Connector/R2020b\"],\"version\":\"1.0\"}"
      mask Help: web("DocumentationServerTrayTL.html")
      mask DialogControl Container6 Prompt: GPU
      mask DialogControl Container7 Prompt: CPU
      mask DialogControl Container9 Prompt: IT Tray
      mask DialogControl Container8 Prompt: Initial Conditions
      mask Display: image('icon_serverPlateTL.png');

== system SimscapeCustomComponents_lib/Datacenter/Utilities ==
  Custom Dynamic Load (3-phase) block : datacenter_lib/Custom Dynamic Load (3-phase) block  Pf=0.98  THD=0  N=10
      settings: InternalSimscapePortConfiguration="{\"Bottom\":[],\"Left\":[{\"id\":\"Pw\",\"label\":\"Pvec\",\"type\":\"input\"}],\"Right\":[{\"id\":\"P\",\"label\":\"P\",\"type\":\"output\"},{\"id\":\"Q\",\"label\":\"Q\",\"type\":\"output\"}],\"Top\":[]}"
  Flow Multiplier : datacenter_lib/Flow Multiplier
      settings: InternalSimscapePortConfiguration="{\"Bottom\":[],\"Left\":[{\"id\":\"A\",\"label\":\"A\",\"type\":\"foundation.thermal_liquid.thermal_liquid\"}],\"Right\":[{\"id\":\"B\",\"label\":\"B\",\"type\":\"foundation.thermal_liquid.thermal_liquid\"}],\"Top\":[{\"id\":\"Na\",\"label\":\"Na\",\"type\":\"input\"},{\"id\":\"Nb\",\"label\":\"Nb\",\"type\":\"input\"}]}"
  Thermal Multiplier : datacenter_lib/Thermal Multiplier
      settings: InternalSimscapePortConfiguration="{\"Bottom\":[],\"Left\":[{\"id\":\"A\",\"label\":\"A\",\"type\":\"foundation.thermal.thermal\"}],\"Right\":[{\"id\":\"B\",\"label\":\"B\",\"type\":\"foundation.thermal.thermal\"}],\"Top\":[{\"id\":\"Na\",\"label\":\"Na\",\"type\":\"input\"},{\"id\":\"Nb\",\"label\":\"Nb\",\"type\":\"input\"}]}"

== system SimscapeCustomComponents_lib/Microgrid and Renewables/Control ==
  BESS : Subsystem
  Generator : Subsystem
  Microgrid : Subsystem
  Renewables : Subsystem
